simulink model "Model_2Systems_IDA"  (R2018b)
settings: Solver=VariableStepAuto  StartTime=0.0  StopTime=10  RelTol=1e-3
values from neighbouring files (symbols this model uses):
  Ts = 0.05; Simulation.Ts = Ts    [Parameters.m]
undefined symbols (not defined in the file or in its folder): p01, p02, q01, q02, Simulation
libraries: simulink x4
settings Model: Creator=oscar  LastModifiedBy=oscar
settings SolverCC: ZeroCrossAlgorithm=Adaptive
settings DataIOCC: OutputOption=SpecifiedOutputTimes  OutputTimes=t_out
settings SFSimCC: SimUseLocalCustomCode=off
settings RTWCC: RTWUseLocalCustomCode=off

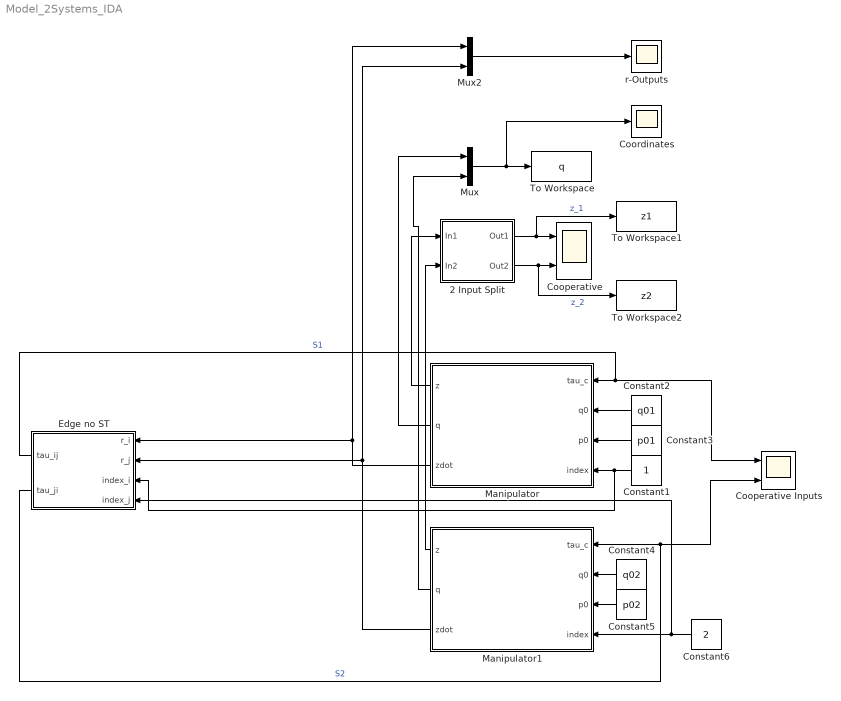
== system Model_2Systems_IDA ==
  2 Input Split : Subsystem
  Constant1 : Constant
  Constant2 : Constant  Value=q01
  Constant3 : Constant  Value=p01
  Constant4 : Constant  Value=q02
  Constant5 : Constant  Value=p02
  Constant6 : Constant  Value=2
  Cooperative : Scope  NumInputPorts=2
  Cooperative Inputs : Scope  NumInputPorts=2
  Coordinates : Scope
  Edge no ST : Subsystem
  Manipulator : Subsystem
  Manipulator1 : Subsystem
  Mux : Mux  Inputs=2
  Mux2 : Mux  Inputs=2
  To Workspace : ToWorkspace  VariableName=q  SaveFormat=Timeseries  SampleTime=-1
  To Workspace1 : ToWorkspace  VariableName=z1  SaveFormat=Timeseries  SampleTime=-1
  To Workspace2 : ToWorkspace  VariableName=z2  SaveFormat=Timeseries  SampleTime=-1
  r-Outputs : Scope
  wires:
  Mux/1 -> Coordinates/1, To Workspace/1
  Manipulator/2(q) -> Mux/1
  Manipulator1/2(q) -> Mux/2
  Constant2/1 -> Manipulator/2(q0)
  Constant3/1 -> Manipulator/3(p0)
  Constant4/1 -> Manipulator1/2(q0)
  Constant5/1 -> Manipulator1/3(p0)
  Edge no ST/1(tau_ij) -> Manipulator/1(tau_c), Cooperative Inputs/1  "S1"
  Edge no ST/2(tau_ji) -> Manipulator1/1(tau_c), Cooperative Inputs/2  "S2"
  Manipulator1/3(zdot) -> Edge no ST/2(r_j), Mux2/2
  Constant1/1 -> Manipulator/4(index), Edge no ST/3(index_i)
  Constant6/1 -> Manipulator1/4(index), Edge no ST/4(index_j)
  Manipulator/3(zdot) -> Edge no ST/1(r_i), Mux2/1
  Mux2/1 -> r-Outputs/1
  Manipulator/1(z) -> 2 Input Split/1(In1)
  Manipulator1/1(z) -> 2 Input Split/2(In2)
  2 Input Split/1(Out1) -> To Workspace1/1, Cooperative/1  "z_1"
  2 Input Split/2(Out2) -> To Workspace2/1, Cooperative/2  "z_2"

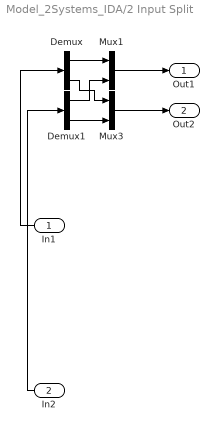
== system Model_2Systems_IDA/2 Input Split ==
  In1 : Inport
  In2 : Inport  Port=2
  Demux : Demux  Outputs=2
  Demux1 : Demux  Outputs=2
  Mux1 : Mux  Inputs=2
  Mux3 : Mux  Inputs=2
  Out1 : Outport
  Out2 : Outport  Port=2
  wires:
  Demux/1 -> Mux1/1
  Mux1/1 -> Out1/1
  In1/1 -> Demux/1
  Demux1/2 -> Mux3/2
  Mux3/1 -> Out2/1
  Demux1/1 -> Mux1/2
  Demux/2 -> Mux3/1
  In2/1 -> Demux1/1

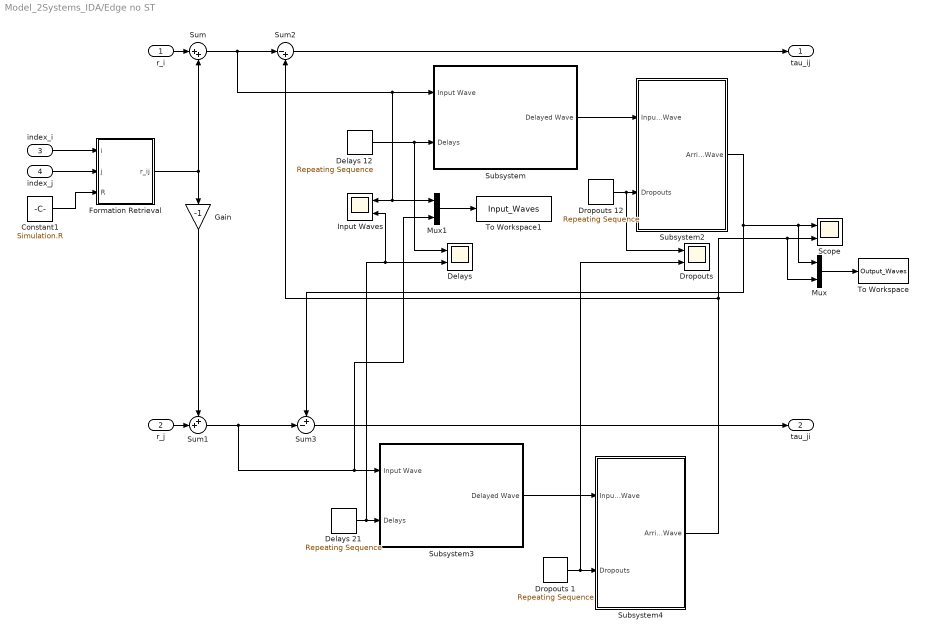
== system Model_2Systems_IDA/Edge no ST ==
  r_i : Inport
  r_j : Inport  Port=2
  index_i : Inport  Port=3
  index_j : Inport  Port=4
  Constant1 : Constant  Value=Simulation.R
  Delays : Scope  NumInputPorts=2
  Delays 12 : simulink/Sources/Repeating Sequence  rep_seq_t=t_delays  rep_seq_y=delays_12
  Delays 21 : simulink/Sources/Repeating Sequence  rep_seq_t=t_delays  rep_seq_y=delays_21
  Dropouts : Scope  NumInputPorts=2
  Dropouts 1 : simulink/Sources/Repeating Sequence  rep_seq_t=t_delays  rep_seq_y=dropouts_21
  Dropouts 12 : simulink/Sources/Repeating Sequence  rep_seq_t=t_delays  rep_seq_y=dropouts_12
  Formation Retrieval : MATLAB Function  TreatAsAtomicUnit=on
  Gain : Gain  Gain=-1
  Input Waves : Scope  NumInputPorts=2
  Mux : Mux  Inputs=2
  Mux1 : Mux  Inputs=2
  Scope : Scope  NumInputPorts=2
  Subsystem : Subsystem
  Subsystem2 : Subsystem
  Subsystem3 : Subsystem
  Subsystem4 : Subsystem
  Sum : Sum  Inputs=|++
  Sum1 : Sum  Inputs=++|
  Sum2 : Sum  Inputs=|-+
  Sum3 : Sum  Inputs=+-|
  To Workspace : ToWorkspace  VariableName=Output_Waves  SaveFormat=Timeseries  SampleTime=-1
  To Workspace1 : ToWorkspace  VariableName=Input_Waves  SaveFormat=Timeseries  SampleTime=-1
  tau_ij : Outport
  tau_ji : Outport  Port=2
  wires:
  r_i/1 -> Sum/1
  r_j/1 -> Sum1/2
  Sum2/1 -> tau_ij/1
  index_i/1 -> Formation Retrieval/1(i)
  index_j/1 -> Formation Retrieval/2(j)
  Formation Retrieval/1(r_ij) -> Gain/1, Sum/2
  Gain/1 -> Sum1/1
  Constant1/1 -> Formation Retrieval/3(R)
  Delays 12/1 -> Delays/1, Subsystem/2(Delays)
  Subsystem/1(Delayed Wave) -> Subsystem2/1(Input Wave)
  Sum3/1 -> tau_ji/1
  Dropouts 12/1 -> Dropouts/1, Subsystem2/2(Dropouts)
  Subsystem2/1(Arriving Wave) -> Sum3/1, Mux/1, Scope/1
  Dropouts 1/1 -> Dropouts/2, Subsystem4/2(Dropouts)
  Mux/1 -> To Workspace/1
  Sum/1 -> Sum2/1, Subsystem/1(Input Wave), Input Waves/1, Mux1/1
  Mux1/1 -> To Workspace1/1
  Sum1/1 -> Mux1/2, Subsystem3/1(Input Wave), Sum3/2
  Delays 21/1 -> Input Waves/2, Delays/2, Subsystem3/2(Delays)
  Subsystem3/1(Delayed Wave) -> Subsystem4/1(Input Wave)
  Subsystem4/1(Arriving Wave) -> Mux/2, Scope/2, Sum2/2

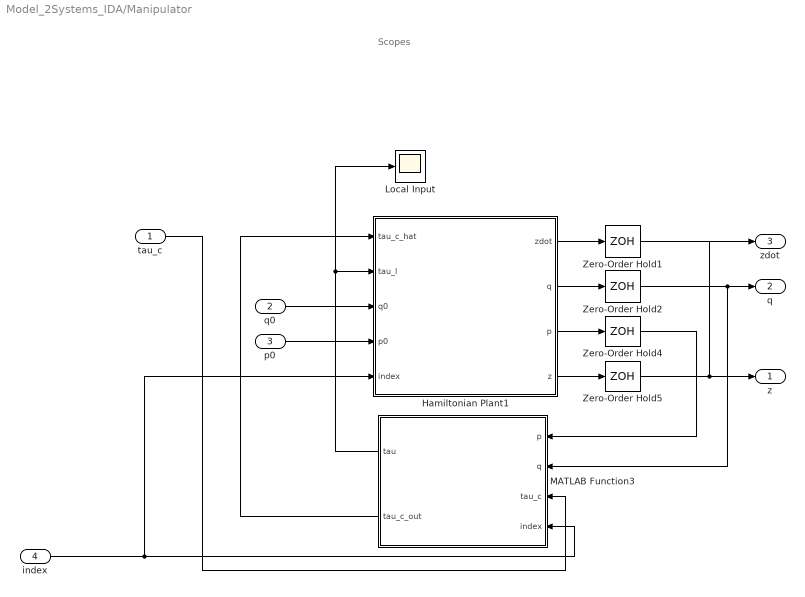
== system Model_2Systems_IDA/Manipulator ==
  note: Scopes
  tau_c : Inport
  q0 : Inport  Port=2
  p0 : Inport  Port=3
  index : Inport  Port=4
  Hamiltonian Plant1 : Subsystem
  Local Input : Scope
  MATLAB Function3 : MATLAB Function  TreatAsAtomicUnit=on
  Zero-Order Hold{1..2,4..5} (4 alike) : ZeroOrderHold  SampleTime=Ts
  z : Outport
  q : Outport  Port=2
  zdot : Outport  Port=3
  wires:
  Hamiltonian Plant1/2(q) -> Zero-Order Hold2/1
  index/1 -> Hamiltonian Plant1/5(index), MATLAB Function3/4(index)
  Hamiltonian Plant1/1(zdot) -> Zero-Order Hold1/1
  MATLAB Function3/1(tau) -> Local Input/1, Hamiltonian Plant1/2(tau_l)
  Hamiltonian Plant1/4(z) -> Zero-Order Hold5/1
  p0/1 -> Hamiltonian Plant1/4(p0)
  Hamiltonian Plant1/3(p) -> Zero-Order Hold4/1
  q0/1 -> Hamiltonian Plant1/3(q0)
  Zero-Order Hold2/1 -> q/1, MATLAB Function3/2(q)
  Zero-Order Hold4/1 -> MATLAB Function3/1(p)
  Zero-Order Hold1/1 -> ?
  Zero-Order Hold5/1 -> zdot/1, z/1
  tau_c/1 -> MATLAB Function3/3(tau_c)
  MATLAB Function3/2(tau_c_out) -> Hamiltonian Plant1/1(tau_c_hat)

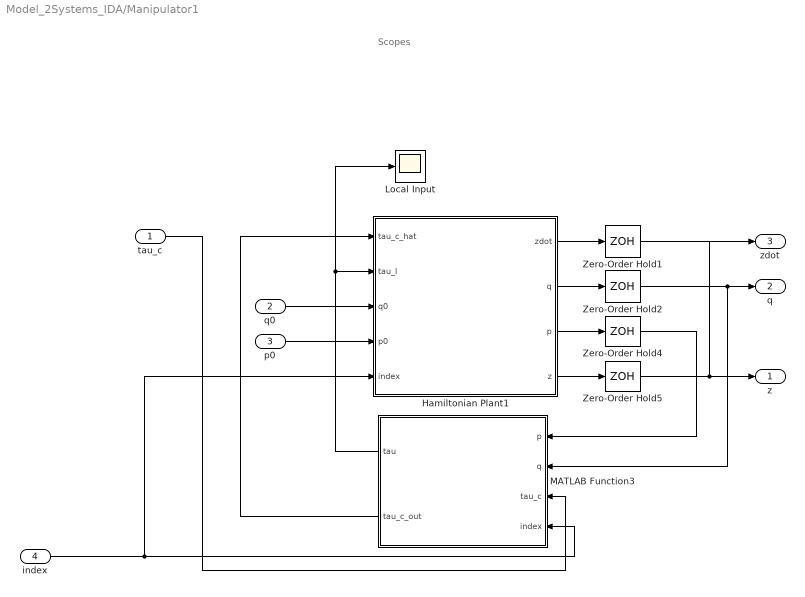
== system Model_2Systems_IDA/Manipulator1 ==
  note: Scopes
  tau_c : Inport
  q0 : Inport  Port=2
  p0 : Inport  Port=3
  index : Inport  Port=4
  Hamiltonian Plant1 : Subsystem
  Local Input : Scope
  MATLAB Function3 : MATLAB Function  TreatAsAtomicUnit=on
  Zero-Order Hold{1..2,4..5} (4 alike) : ZeroOrderHold  SampleTime=Ts
  z : Outport
  q : Outport  Port=2
  zdot : Outport  Port=3
  wires:
  Hamiltonian Plant1/2(q) -> Zero-Order Hold2/1
  index/1 -> Hamiltonian Plant1/5(index), MATLAB Function3/4(index)
  Hamiltonian Plant1/1(zdot) -> Zero-Order Hold1/1
  MATLAB Function3/1(tau) -> Local Input/1, Hamiltonian Plant1/2(tau_l)
  Hamiltonian Plant1/4(z) -> Zero-Order Hold5/1
  p0/1 -> Hamiltonian Plant1/4(p0)
  Hamiltonian Plant1/3(p) -> Zero-Order Hold4/1
  q0/1 -> Hamiltonian Plant1/3(q0)
  Zero-Order Hold2/1 -> q/1, MATLAB Function3/2(q)
  Zero-Order Hold4/1 -> MATLAB Function3/1(p)
  Zero-Order Hold1/1 -> ?
  Zero-Order Hold5/1 -> zdot/1, z/1
  tau_c/1 -> MATLAB Function3/3(tau_c)
  MATLAB Function3/2(tau_c_out) -> Hamiltonian Plant1/1(tau_c_hat)

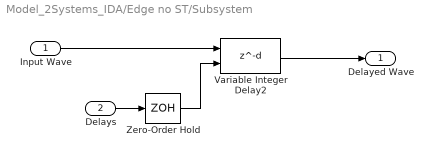
== system Model_2Systems_IDA/Edge no ST/Subsystem ==
  Input Wave : Inport
  Delays : Inport  Port=2
  Variable Integer Delay2 : Delay  DelayLengthSource=Input port  PreventDirectFeedthrough=on  SampleTime=Ts
      settings: InputPortMap=u0,p1
  Zero-Order Hold : ZeroOrderHold  SampleTime=Ts
  Delayed Wave : Outport
  wires:
  Input Wave/1 -> Variable Integer Delay2/1
  Variable Integer Delay2/1 -> Delayed Wave/1
  Delays/1 -> Zero-Order Hold/1
  Zero-Order Hold/1 -> Variable Integer Delay2/2

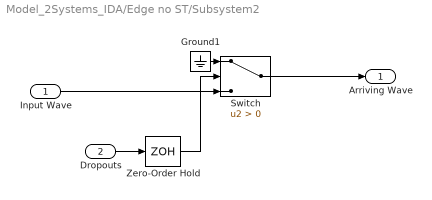
== system Model_2Systems_IDA/Edge no ST/Subsystem2 ==
  Input Wave : Inport
  Dropouts : Inport  Port=2
  Ground1 : Ground
  Switch : Switch  Criteria=u2 > Threshold
  Zero-Order Hold : ZeroOrderHold  SampleTime=Ts
  Arriving Wave : Outport
  wires:
  Input Wave/1 -> Switch/3
  Switch/1 -> Arriving Wave/1
  Dropouts/1 -> Zero-Order Hold/1
  Zero-Order Hold/1 -> Switch/2
  Ground1/1 -> Switch/1

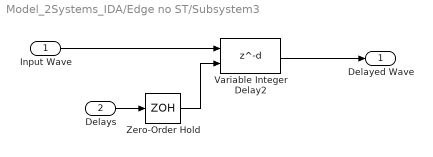
== system Model_2Systems_IDA/Edge no ST/Subsystem3 ==
  Input Wave : Inport
  Delays : Inport  Port=2
  Variable Integer Delay2 : Delay  DelayLengthSource=Input port  PreventDirectFeedthrough=on  SampleTime=Ts
      settings: InputPortMap=u0,p1
  Zero-Order Hold : ZeroOrderHold  SampleTime=Ts
  Delayed Wave : Outport
  wires:
  Input Wave/1 -> Variable Integer Delay2/1
  Variable Integer Delay2/1 -> Delayed Wave/1
  Delays/1 -> Zero-Order Hold/1
  Zero-Order Hold/1 -> Variable Integer Delay2/2

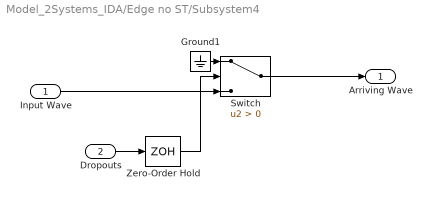
== system Model_2Systems_IDA/Edge no ST/Subsystem4 ==
  Input Wave : Inport
  Dropouts : Inport  Port=2
  Ground1 : Ground
  Switch : Switch  Criteria=u2 > Threshold
  Zero-Order Hold : ZeroOrderHold  SampleTime=Ts
  Arriving Wave : Outport
  wires:
  Input Wave/1 -> Switch/3
  Switch/1 -> Arriving Wave/1
  Dropouts/1 -> Zero-Order Hold/1
  Zero-Order Hold/1 -> Switch/2
  Ground1/1 -> Switch/1

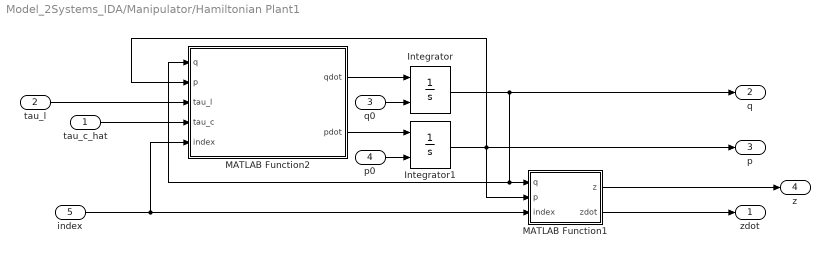
== system Model_2Systems_IDA/Manipulator/Hamiltonian Plant1 ==
  tau_c_hat : Inport
  tau_l : Inport  Port=2
  q0 : Inport  Port=3
  p0 : Inport  Port=4
  index : Inport  Port=5
  Integrator : Integrator  InitialConditionSource=external  InitialCondition=q01
  Integrator1 : Integrator  InitialConditionSource=external  InitialCondition=p02
  MATLAB Function1 : MATLAB Function  TreatAsAtomicUnit=on
  MATLAB Function2 : MATLAB Function  TreatAsAtomicUnit=on
  zdot : Outport
  q : Outport  Port=2
  p : Outport  Port=3
  z : Outport  Port=4
  wires:
  tau_l/1 -> MATLAB Function2/3(tau_l)
  MATLAB Function2/2(pdot) -> Integrator1/1
  Integrator1/1 -> MATLAB Function2/2(p), p/1, MATLAB Function1/2(p)
  Integrator/1 -> q/1, MATLAB Function2/1(q), MATLAB Function1/1(q)
  MATLAB Function2/1(qdot) -> Integrator/1
  p0/1 -> Integrator1/2
  q0/1 -> Integrator/2
  MATLAB Function1/1(z) -> z/1
  index/1 -> MATLAB Function1/3(index), MATLAB Function2/5(index)
  tau_c_hat/1 -> MATLAB Function2/4(tau_c)
  MATLAB Function1/2(zdot) -> zdot/1

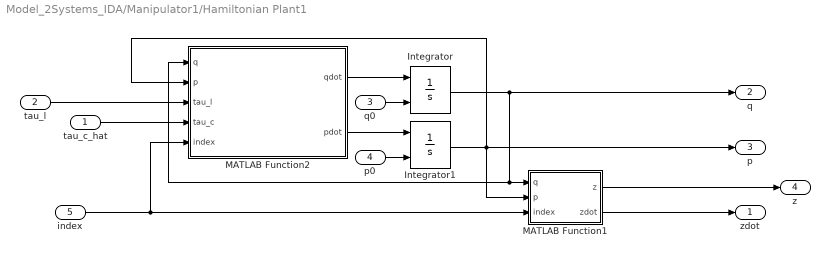
== system Model_2Systems_IDA/Manipulator1/Hamiltonian Plant1 ==
  tau_c_hat : Inport
  tau_l : Inport  Port=2
  q0 : Inport  Port=3
  p0 : Inport  Port=4
  index : Inport  Port=5
  Integrator : Integrator  InitialConditionSource=external  InitialCondition=q01
  Integrator1 : Integrator  InitialConditionSource=external  InitialCondition=p02
  MATLAB Function1 : MATLAB Function  TreatAsAtomicUnit=on
  MATLAB Function2 : MATLAB Function  TreatAsAtomicUnit=on
  zdot : Outport
  q : Outport  Port=2
  p : Outport  Port=3
  z : Outport  Port=4
  wires:
  tau_l/1 -> MATLAB Function2/3(tau_l)
  MATLAB Function2/2(pdot) -> Integrator1/1
  Integrator1/1 -> MATLAB Function2/2(p), p/1, MATLAB Function1/2(p)
  Integrator/1 -> q/1, MATLAB Function2/1(q), MATLAB Function1/1(q)
  MATLAB Function2/1(qdot) -> Integrator/1
  p0/1 -> Integrator1/2
  q0/1 -> Integrator/2
  MATLAB Function1/1(z) -> z/1
  index/1 -> MATLAB Function1/3(index), MATLAB Function2/5(index)
  tau_c_hat/1 -> MATLAB Function2/4(tau_c)
  MATLAB Function1/2(zdot) -> zdot/1

== matlab function Model_2Systems_IDA/Manipulator1/Hamiltonian Plant1/MATLAB Function1 ==
  data: q input; z output; p input; zdot output; index input
function [z, zdot] = toz(q, p, index)

    coder.extrinsic('Manipulator_IDAz');
    z = zeros(2, 1);
    zdot = zeros(2, 1);
    [z, zdot] = Manipulator_IDAz(q, p, index);

== matlab function Model_2Systems_IDA/Manipulator1/Hamiltonian Plant1/MATLAB Function2 ==
  data: q input; qdot output; p input; tau_l input; pdot output; tau_c input; index input
function [qdot, pdot] = fcn(q, p, tau_l, tau_c, index)

    coder.extrinsic('Manipulator_IDADynamics');
    qdot = zeros(3, 1);
    pdot = zeros(3, 1);
    [qdot, pdot] = Manipulator_IDADynamics(q, p, tau_l, tau_c, index);

== matlab function Model_2Systems_IDA/Manipulator1/MATLAB Function3 ==
  data: p input; q input; tau_c input; tau output; index input; tau_c_out output
function [tau, tau_c_out]  = LocalControl(p, q, tau_c, index)
    

coder.extrinsic('Manipulator_IDAControl');
tau = zeros(3, 1);
tau_c_out = zeros(2, 1);
[tau, tau_c_out] = Manipulator_IDAControl(q, p, tau_c, index);

== matlab function Model_2Systems_IDA/Edge no ST/Formation Retrieval ==
  data: i input; r_ij output; j input; R input
function r_ij = get_rij(i, j, R)
    %r_ij = zeros(2,1);
    r_ij = [R((i - 1)*2 + 1, j);R(2*i, j)];
end

== matlab function Model_2Systems_IDA/Manipulator/Hamiltonian Plant1/MATLAB Function1 ==
  data: q input; z output; p input; zdot output; index input
function [z, zdot] = toz(q, p, index)

    coder.extrinsic('Manipulator_IDAz');
    z = zeros(2, 1);
    zdot = zeros(2, 1);
    [z, zdot] = Manipulator_IDAz(q, p, index);

== matlab function Model_2Systems_IDA/Manipulator/Hamiltonian Plant1/MATLAB Function2 ==
  data: q input; qdot output; p input; tau_l input; pdot output; tau_c input; index input
function [qdot, pdot] = fcn(q, p, tau_l, tau_c, index)

    coder.extrinsic('Manipulator_IDADynamics');
    qdot = zeros(3, 1);
    pdot = zeros(3, 1);
    [qdot, pdot] = Manipulator_IDADynamics(q, p, tau_l, tau_c, index);

== matlab function Model_2Systems_IDA/Manipulator/MATLAB Function3 ==
  data: p input; q input; tau_c input; tau output; index input; tau_c_out output
function [tau, tau_c_out]  = LocalControl(p, q, tau_c, index)
    

coder.extrinsic('Manipulator_IDAControl');
tau = zeros(3, 1);
tau_c_out = zeros(2, 1);
[tau, tau_c_out] = Manipulator_IDAControl(q, p, tau_c, index);
